simulink model "Copy_of_provaHITL_12_10_completosensori_BUONO"  (R2020b)
settings: Solver=FixedStepDiscrete  StartTime=0.0  StopTime=Inf  FixedStep=0.02  RelTol=1e-3  EnableMultiTasking=on
PostLoadFcn:
  | , if any(exist('dsrtsu_mdlpostloadfcn', 'file') == [2, 3, 6]), try dsrtsu_mdlpostloadfcn('Execute', bdroot); catch fprintf('Error in PostLoadFcn (dsrtsu_mdlpostloadfcn) for model "%s":\n %s\n', bdroot, lasterr); end, end,
InitFcn:
  | , if any(exist('rtifpga_mdlclblib', 'file') ~= 0), rtifpga_mdlclblib('Init', bdroot); end,
values from neighbouring files (symbols this model uses):
  attuatore_Amax = deg2rad(27)    [AVVIO_AENEA_DATA.m]    (also in workspace_SFT.mat = 0.349065850399)
  attuatore_Amin = deg2rad(-23)    [AVVIO_AENEA_DATA.m]
  attuatore_Emax = deg2rad(18)    [AVVIO_AENEA_DATA.m]    (also in workspace_SFT.mat = 0.436332312999)
  attuatore_Emin = deg2rad(-32)    [AVVIO_AENEA_DATA.m]
  attuatore_Rmax = deg2rad(30)    [AVVIO_AENEA_DATA.m]    (also in workspace_SFT.mat = 0.436332312999)
  attuatore_Rmin = deg2rad(-30)    [AVVIO_AENEA_DATA.m]
  attuatore_Tmax = 1    [AVVIO_AENEA_DATA.m]    (also in workspace_SFT.mat = 0.6)
  attuatore_Tmin = 0    [AVVIO_AENEA_DATA.m]    (also in workspace_SFT.mat)
  interventoA_05 = 6    [AVVIO_AENEA_DATA.m]    (also in workspace_SFT.mat)
  interventoA_1 = 2    [AVVIO_AENEA_DATA.m]    (also in workspace_SFT.mat)
  interventoE_05 = 7.5    [AVVIO_AENEA_DATA.m]    (also in workspace_SFT.mat)
  interventoE_1 = 3.2    [AVVIO_AENEA_DATA.m]    (also in workspace_SFT.mat)
  interventoT = 0.1    [AVVIO_AENEA_DATA.m]    (also in workspace_SFT.mat)
  inv_A = -1    [AVVIO_AENEA_DATA.m]
  inv_comp_h = -1    [AVVIO_AENEA_DATA.m]
  inv_E = 1    [AVVIO_AENEA_DATA.m]
  inv_R = 1    [AVVIO_AENEA_DATA.m]
  inv_T = 1    [AVVIO_AENEA_DATA.m]
  K_AW_B_AP_quota = 1000    [AVVIO_AENEA_DATA.m]
  K_AW_B_becc = -250    [AVVIO_AENEA_DATA.m]
  K_AW_B_imb = 0    [AVVIO_AENEA_DATA.m]
  K_AW_B_roll = 500    [AVVIO_AENEA_DATA.m]
  K_imb_inv = -0.001306    [AVVIO_AENEA_DATA.m]
  Kd_h_app = 0.085    [AVVIO_AENEA_DATA.m]
  Kd_h_flare = 0.01    [AVVIO_AENEA_DATA.m]
  Ki_AP_quota_select = 0.01936    [AVVIO_AENEA_DATA.m]
  Ki_AP_rotta = 0.002    [AVVIO_AENEA_DATA.m]
  Ki_AP_vel = 0.025175    [AVVIO_AENEA_DATA.m]
  Ki_becch = -0.1963    [AVVIO_AENEA_DATA.m]
  Ki_h_app = 0.055    [AVVIO_AENEA_DATA.m]
  Ki_h_cruise = 0.008    [AVVIO_AENEA_DATA.m]
  Ki_h_flare = 0.07    [AVVIO_AENEA_DATA.m]
  Ki_roll = 0.004528    [AVVIO_AENEA_DATA.m]
  Kp_AP_quota_hold_h = 0.5503    [AVVIO_AENEA_DATA.m]
  Kp_AP_quota_hold_l = 0.5503    [AVVIO_AENEA_DATA.m]
  Kp_AP_quota_select = 0.02647    [AVVIO_AENEA_DATA.m]
  Kp_AP_rotta = 0.520    (= 0.52)    [AVVIO_AENEA_DATA.m]
  Kp_AP_vel = 0.132175    [AVVIO_AENEA_DATA.m]
  Kp_becch = -0.30    (= -0.3)    [AVVIO_AENEA_DATA.m]
  Kp_comp_h = 0.035    [AVVIO_AENEA_DATA.m]
  Kp_h_app_max = 0.086    [AVVIO_AENEA_DATA.m]
  Kp_h_app_min = 0.01    [AVVIO_AENEA_DATA.m]
  Kp_h_cruise = 0.04    [AVVIO_AENEA_DATA.m]
  Kp_h_flare = 0.1    [AVVIO_AENEA_DATA.m]
  Kp_imb = 0.0019415    [AVVIO_AENEA_DATA.m]
  Kp_p = 0.006913    [AVVIO_AENEA_DATA.m]
  Kp_q = -0.025    [AVVIO_AENEA_DATA.m]
  Kp_roll = 0.0718    [AVVIO_AENEA_DATA.m]
  Kp_Rotta_ATO = 4    [AVVIO_AENEA_DATA.m]    (also in workspace_SFT.mat)
  phi_max = deg2rad(30)    [AVVIO_AENEA_DATA.m]
  phi_min = deg2rad(-30)    [AVVIO_AENEA_DATA.m]
  safe_phi = 55    [AVVIO_AENEA_DATA.m]    (also in workspace_SFT.mat)
  safe_V = 40    [AVVIO_AENEA_DATA.m]    (also in workspace_SFT.mat)
  t_AP = 0.02    [AVVIO_AENEA_DATA.m]    (also in workspace_SFT.mat)
  theta_max = deg2rad(15)    [AVVIO_AENEA_DATA.m]
  theta_min = deg2rad(-15)    [AVVIO_AENEA_DATA.m]
  time_alarm_SAFE = 1    [AVVIO_AENEA_DATA.m]    (also in workspace_SFT.mat)
  tsamp = 0.02    [workspace_SFT.mat]
  V_max = 30    [AVVIO_AENEA_DATA.m]
  V_stall = 11    [AVVIO_AENEA_DATA.m]
  vel_wp1_al = 25    [AVVIO_AENEA_DATA.m]    (also in workspace_SFT.mat)
  vel_wp2_al = 20    [AVVIO_AENEA_DATA.m]    (also in workspace_SFT.mat)
undefined symbols (not defined in the file or in its folder): DiscIntNeverNeededParam, Newton, Raphson
libraries: simulink_extras x33, arduinolib x20, pid_lib x8, svdutilitieslib x3, simulink x3, dspsigops x3, aerolibtransform2sys x2, aerolibtransform2 x2
(part 5 of 8)

== system Copy_of_provaHITL_12_10_completosensori_BUONO/AUTOPILOTA/CONTROLLI INTERNI E SWITCH1/Controllore PID/elevator - landing ==
  In1 : Inport
  Tas : Inport  Port=2
  AL : Inport  Port=3
  Constant5 : Constant  Value=0
  Multiport Switch2 : MultiPortSwitch  DataPortOrder=Zero-based contiguous  Inputs=2  zeroidx=on
  Switch1 : Switch  Threshold=16
  Out1 : Outport  VectorParamsAs1DForOutWhenUnconnected=off
  wires:
  Multiport Switch2/1 -> Out1/1
  Tas/1 -> Switch1/2
  In1/1 -> Multiport Switch2/2, Switch1/1
  AL/1 -> Multiport Switch2/1
  Constant5/1 -> Switch1/3
  Switch1/1 -> Multiport Switch2/3

== system Copy_of_provaHITL_12_10_completosensori_BUONO/AUTOPILOTA/CONTROLLI INTERNI E SWITCH1/Controllore PID/elevator - takeoff ==
  In1 : Inport
  Fase_ATO : Inport  Port=2
  ATO : Inport  Port=3
  eq_rot : Inport  Port=4
  Degrees to Radians : simulink_extras/Transformations/Degrees to Radians
  Multiport Switch1 : MultiPortSwitch  DataPortOrder=Zero-based contiguous  Inputs=5  zeroidx=on
  Multiport Switch2 : MultiPortSwitch  DataPortOrder=Zero-based contiguous  Inputs=2  zeroidx=on
  Out1 : Outport  VectorParamsAs1DForOutWhenUnconnected=off
  wires:
  ATO/1 -> Multiport Switch2/1
  In1/1 -> Multiport Switch1/6, Multiport Switch1/5, Multiport Switch2/2
  Multiport Switch2/1 -> Out1/1
  Multiport Switch1/1 -> Multiport Switch2/3
  Fase_ATO/1 -> Multiport Switch1/1
  eq_rot/1 -> Degrees to Radians/1
  Degrees to Radians/1 -> Multiport Switch1/4, Multiport Switch1/3, Multiport Switch1/2

== system Copy_of_provaHITL_12_10_completosensori_BUONO/AUTOPILOTA/GESTIONE AUTOPILOTI1/Interruttore_Intervento/Enabled Subsystem ==
  Time : Inport
  Enable : EnablePort
  Constant1 : Constant  Value=0
  Constant2 : Constant
  Switch : Switch  Criteria=u2 > Threshold  Threshold=2
  1/0 : Outport  VectorParamsAs1DForOutWhenUnconnected=off
  wires:
  Time/1 -> Switch/2
  Constant1/1 -> Switch/1
  Constant2/1 -> Switch/3
  Switch/1 -> 1/0/1

== system Copy_of_provaHITL_12_10_completosensori_BUONO/AUTOPILOTA/GESTIONE AUTOPILOTI1/Interruttore_Intervento/Resettable Subsystem ==
  Reset : ResetPort  DisableCoverage=on
  CLOCK : Subsystem
  Time : Outport  VectorParamsAs1DForOutWhenUnconnected=off
  wires:
  CLOCK/1(Time) -> Time/1

== system Copy_of_provaHITL_12_10_completosensori_BUONO/AUTOPILOTA/GESTIONE AUTOPILOTI1/Interruttore_Safe/Enabled Subsystem ==
  Time : Inport
  Enable : EnablePort
  Constant1 : Constant  Value=0
  Constant2 : Constant
  Switch : Switch  Criteria=u2 > Threshold  Threshold=2
  1/0 : Outport  VectorParamsAs1DForOutWhenUnconnected=off
  wires:
  Time/1 -> Switch/2
  Constant1/1 -> Switch/1
  Constant2/1 -> Switch/3
  Switch/1 -> 1/0/1

== system Copy_of_provaHITL_12_10_completosensori_BUONO/AUTOPILOTA/GESTIONE AUTOPILOTI1/Interruttore_Safe/Resettable Subsystem ==
  Reset : ResetPort  DisableCoverage=on
  CLOCK : Subsystem
  Time : Outport  VectorParamsAs1DForOutWhenUnconnected=off
  wires:
  CLOCK/1(Time) -> Time/1

== system Copy_of_provaHITL_12_10_completosensori_BUONO/AUTOPILOTA/GESTIONE AUTOPILOTI1/Intervento Manager/Alarm_Timing_0.5sec ==
  Intervento_IN : Inport
  "Enabled " : Subsystem  TreatAsAtomicUnit=on
  Resettable Subsystem : Subsystem  TreatAsAtomicUnit=on
  Alarm : Outport  VectorParamsAs1DForOutWhenUnconnected=off
  wires:
  Intervento_IN/1 -> Resettable Subsystem/Reset, "Enabled "/Enable
  Resettable Subsystem/1(Time) -> "Enabled "/1("Time ")
  "Enabled "/1(Alarm_Int) -> Alarm/1

== system Copy_of_provaHITL_12_10_completosensori_BUONO/AUTOPILOTA/GESTIONE AUTOPILOTI1/Intervento Manager/Alarm_Timing_1sec ==
  Intervento_IN : Inport
  "Enabled " : Subsystem  TreatAsAtomicUnit=on
  Resettable Subsystem : Subsystem  TreatAsAtomicUnit=on
  Alarm : Outport  VectorParamsAs1DForOutWhenUnconnected=off
  wires:
  Intervento_IN/1 -> Resettable Subsystem/Reset, "Enabled "/Enable
  Resettable Subsystem/1(Time) -> "Enabled "/1("Time ")
  "Enabled "/1(Alarm_Int) -> Alarm/1

== system Copy_of_provaHITL_12_10_completosensori_BUONO/AUTOPILOTA/GESTIONE AUTOPILOTI1/Safe Manager/Alarm_Timing ==
  Alarm_IN : Inport
  "Enabled " : Subsystem  TreatAsAtomicUnit=on
  Resettable Subsystem : Subsystem  TreatAsAtomicUnit=on
  Alarm : Outport  VectorParamsAs1DForOutWhenUnconnected=off
  wires:
  Alarm_IN/1 -> Resettable Subsystem/Reset, "Enabled "/Enable
  Resettable Subsystem/1(Time) -> "Enabled "/1("Time ")
  "Enabled "/1(Alarm Safe) -> Alarm/1

== system Copy_of_provaHITL_12_10_completosensori_BUONO/AUTOPILOTA/Subsystem1/Subsystem1/APPROACH ==
  dist : Inport
  h_g : Inport  Port=2
  x_g : Inport  Port=3
  V_ : Inport  Port=4
  Enable : EnablePort  ShowOutputPort=on
  Abs : Abs
  Atan : Trigonometry  Operator=atan
  Constant1 : Constant  Value=20  SampleTime=0.02
  Constant2 : Constant  SampleTime=0.02
  Constant3 : Constant  SampleTime=0.02
  Constant4 : Constant  Value=0  SampleTime=0.02
  Discrete-Time Integrator : DiscreteIntegrator  gainval=1  ExternalReset=rising  SampleTime=0.02  LimitOutput=on  UpperSaturationLimit=1  LowerSaturationLimit=0  ICPrevOutput=DiscIntNeverNeededParam  ICPrevScaledInput=DiscIntNeverNeededParam
  Divide : Product  Inputs=*/
  Gain : Gain  Gain=-1
  MATLAB Function : MATLAB Function  TreatAsAtomicUnit=on
  Multiply : Product
  Multiply1 : Product
  Mux : Mux
  Sum : Sum  Inputs=|+-
  Sum1 : Sum  Inputs=|+-
  Switch : Switch  Criteria=u2 > Threshold
  x_g0 : Constant  Value=-100  SampleTime=0.02
  h_ref : Outport  VectorParamsAs1DForOutWhenUnconnected=off
  V1 : Outport  Port=2  VectorParamsAs1DForOutWhenUnconnected=off
  flare_data : Outport  Port=3  VectorParamsAs1DForOutWhenUnconnected=off
  landing_abort : Outport  Port=4  VectorParamsAs1DForOutWhenUnconnected=off
  rc_ref_app : Outport  Port=5  VectorParamsAs1DForOutWhenUnconnected=off
  wires:
  Constant1/1 -> V1/1
  h_g/1 -> Divide/1
  Sum/1 -> Divide/2
  x_g/1 -> Sum/1
  Sum1/1 -> Gain/1
  Gain/1 -> Multiply/2
  dist/1 -> Sum1/1
  x_g0/1 -> Sum/2, MATLAB Function/3(xg0), Sum1/2
  Multiply/1 -> h_ref/1
  Mux/1 -> flare_data/1
  MATLAB Function/2(h_f_out) -> Mux/2
  MATLAB Function/1(x_f_out) -> Mux/1
  Abs/1 -> MATLAB Function/2(gamma)
  MATLAB Function/3(k_x_out) -> Mux/3
  MATLAB Function/4(h_c_out) -> Mux/4
  MATLAB Function/5(no_solution) -> landing_abort/1
  Constant2/1 -> Discrete-Time Integrator/1
  Constant3/1 -> Switch/1
  Enable/1 -> Discrete-Time Integrator/2
  Constant4/1 -> Switch/3
  Discrete-Time Integrator/1 -> Switch/2
  Switch/1 -> MATLAB Function/1(reset)
  V_/1 -> Multiply1/1
  Multiply1/1 -> rc_ref_app/1
  Divide/1 -> Multiply1/2, Multiply/1, Atan/1
  Atan/1 -> Abs/1

== system Copy_of_provaHITL_12_10_completosensori_BUONO/AUTOPILOTA/Subsystem1/Subsystem1/CREAZIONE_WAYPOINT  ==
  Lat_Home : Inport
  Long_Home : Inport  Port=2
  h_Home : Inport  Port=3
  psi_Home : Inport  Port=4
  AUTOLANDING_WAYPOINTS : MATLAB Function  TreatAsAtomicUnit=on
  Constant : Constant  Value=vel_wp1_al
  Constant1 : Constant  Value=vel_wp2_al
  MATLAB Function : MATLAB Function  TreatAsAtomicUnit=on
  Radians to Degrees : simulink_extras/Transformations/Radians to Degrees
  Radians to Degrees1 : simulink_extras/Transformations/Radians to Degrees
  alt waypoint virtuale : Constant  Value=[45 45 45]
  distance waypoints virtuale : Constant  Value=[-1000 -800 2000]
  WP_info : Outport  VectorParamsAs1DForOutWhenUnconnected=off
  WP_param : Outport  Port=2  VectorParamsAs1DForOutWhenUnconnected=off
  wires:
  alt waypoint virtuale/1 -> AUTOLANDING_WAYPOINTS/4(alt)
  distance waypoints virtuale/1 -> MATLAB Function/4(distance)
  Lat_Home/1 -> MATLAB Function/1(lat_ini)
  Long_Home/1 -> MATLAB Function/2(long_ini)
  psi_Home/1 -> MATLAB Function/3(heading)
  h_Home/1 -> AUTOLANDING_WAYPOINTS/3(h_Home)
  MATLAB Function/1(lat_end) -> Radians to Degrees/1
  MATLAB Function/2(long_end) -> Radians to Degrees1/1
  Radians to Degrees/1 -> AUTOLANDING_WAYPOINTS/1(Lat_Home)
  Radians to Degrees1/1 -> AUTOLANDING_WAYPOINTS/2(Long_Home)
  AUTOLANDING_WAYPOINTS/1(WP_info) -> WP_info/1
  AUTOLANDING_WAYPOINTS/2(WP_param) -> WP_param/1
  Constant/1 -> AUTOLANDING_WAYPOINTS/5(vel_wp1_al)
  Constant1/1 -> AUTOLANDING_WAYPOINTS/6(vel_wp2_al)

== system Copy_of_provaHITL_12_10_completosensori_BUONO/AUTOPILOTA/Subsystem1/Subsystem1/FLARE ==
  x_e : Inport
  flare_data : Inport  Port=2
  V_ : Inport  Port=3
  Enable : EnablePort
  Constant1 : Constant  Value=18  SampleTime=0.02
  Demux : Demux
  Exp : Math  SignedPower=on  SaturateOnIntegerOverflow=on
  Exp1 : Math  SignedPower=on  SaturateOnIntegerOverflow=on
  Gain : Gain  Gain=-1
  Gain1 : Gain  Gain=-1
  Gain2 : Gain  Gain=-1
  MATLAB Function : MATLAB Function  Commented=on  TreatAsAtomicUnit=on
  Multiply{,1..3} (4 alike) : Product
  Multiply4 : Product  Inputs=3
  Sum{,1,3..4} (4 alike) : Sum  Inputs=|+-
  Sum2 : Sum  Inputs=|++
  x_e1 : InportShadow
  Tas_ref1 : Outport  VectorParamsAs1DForOutWhenUnconnected=off
  h_ref : Outport  Port=2  VectorParamsAs1DForOutWhenUnconnected=off
  RC_ref : Outport  Port=3  VectorParamsAs1DForOutWhenUnconnected=off
  wires:
  MATLAB Function/1(rotta) -> ?
  Constant1/1 -> Tas_ref1/1
  x_e/1 -> Sum/1
  Sum/1 -> Multiply/1
  Multiply/1 -> Gain/1
  Gain/1 -> Exp/1
  Exp/1 -> Multiply1/1
  Sum1/1 -> Multiply1/2
  Multiply1/1 -> Sum2/1
  flare_data/1 -> Demux/1
  Sum2/1 -> h_ref/1
  Gain1/1 -> Exp1/1
  Demux/1 -> Sum3/2, Sum/2  "x_f"
  Demux/2 -> Sum4/1, Sum1/1  "h_f"
  x_e1/1 -> Sum3/1
  Exp1/1 -> Multiply3/1
  Gain2/1 -> RC_ref/1
  Demux/4 -> Sum4/2, Sum1/2, Sum2/2  "h_c"
  Multiply2/1 -> Gain1/1
  Sum3/1 -> Multiply2/1
  Demux/3 -> Multiply2/2, Multiply4/3, Multiply/2  "k_x"
  Multiply3/1 -> Gain2/1
  Sum4/1 -> Multiply4/1
  V_/1 -> Multiply4/2
  Multiply4/1 -> Multiply3/2

== system Copy_of_provaHITL_12_10_completosensori_BUONO/AUTOPILOTA/Subsystem1/Subsystem1/INSEGUIMENTO CENTRO PISTA ==
  y_e : Inport
  psi_home : Inport  Port=2
  Enable : EnablePort
  Gain1 : Gain
  PID Controller : pid_lib/PID Controller  Controller=PI  Form=Parallel  TimeDomain=Discrete-time  UseExternalTs=off  SampleTime=-1  IntegratorMethod=Forward Euler  FilterMethod=Forward Euler  ControllerParametersSource=external  P=1  I=1  D=0  UseFilter=on  N=100  TunerSelectOption=Transfer Function Based (PID Tuner App)  InitialConditionSource=internal  InitialConditionForIntegrator=0  InitialConditionForFilter=0  DifferentiatorICPrevScaledInput=0  ExternalReset=none  TrackingMode=off  Kt=1  LimitOutput=off  SatLimitsSource=internal  UpperSaturationLimit=inf  LowerSaturationLimit=-inf  LinearizeAsGain=on  AntiWindupMode=none  Kb=1  POutMin=[]  POutMax=[]  IOutMin=[]  IOutMax=[]  DOutMin=[]  DOutMax=[]  NOutMin=[]  NOutMax=[]  SumOutMin=[]  SumOutMax=[]  SaturationOutMin=[]  SaturationOutMax=[]  PParamMin=[]  PParamMax=[]  IParamMin=[]  IParamMax=[]  DParamMin=[]  DParamMax=[]  NParamMin=[]  NParamMax=[]  KbParamMin=[]  KbParamMax=[]  KtParamMin=[]  KtParamMax=[]  KbOutMin=[]  KbOutMax=[]  KtOutMin=[]  KtOutMax=[]  IntegratorOutMin=[]  IntegratorOutMax=[]  FilterOutMin=[]  FilterOutMax=[]  SumI1OutMin=[]  SumI1OutMax=[]  SumI2OutMin=[]  SumI2OutMax=[]  SumI3OutMin=[]  SumI3OutMax=[]  SumI4OutMin=[]  SumI4OutMax=[]  SumDOutMin=[]  SumDOutMax=[]  DifferentiatorOutMin=[]  DifferentiatorOutMax=[]  FilterDiffOutCoefMin=[]  FilterDiffOutCoefMax=[]  ReciprocalOutMin=[]  ReciprocalOutMax=[]  SumDenOutMin=[]  SumDenOutMax=[]  SumNumOutMin=[]  SumNumOutMax=[]  DivideOutMin=[]  DivideOutMax=[]  UdiffTsProdOutMin=[]  UdiffTsProdOutMax=[]  NTsProdOutMin=[]  NTsProdOutMax=[]  UintegralTsProdOutMin=[]  UintegralTsProdOutMax=[]  UngainTsProdOutMin=[]  UngainTsProdOutMax=[]  IntegratorContinuousStateAttributes=''  IntegratorStateMustResolveToSignalObject=off  IntegratorRTWStateStorageClass=Auto  FilterContinuousStateAttributes=''  FilterStateMustResolveToSignalObject=off  FilterRTWStateStorageClass=Auto  ParallelPVariant=ExternalParameters  IdealPVariant=Disabled  IVariant=ExternalParameters  DVariant=Disabled  IntegratorVariant=Discrete  SatVariant=Disabled  AWVariant=Passthrough  PCopyVariant=Disabled  TRVariant=Disabled  FdbkBlocksVariant=Forward  IdealPFdbkVariant=Disabled  SatFdbkVariant=Disabled  DerivativeFilterVariant=Disabled  NVariant=Disabled  NCopyVariant=Disabled_SignalSpec  FilterICVariant=Disabled  IntegratorICVariant=InternalICs  ExternalResetVariant=Disabled  TRSumVariant=Passthrough  SumFdbkVariant=Disabled  SumVariant=Sum_PI  TsampFilterVariant=InternalTs  TsampNgainVariant=Passthrough  TsampIntegralVariant=Passthrough  ExternalSaturationOutDataTypeStr=Inherit: Same as second input
  Radians to Degrees2 : simulink_extras/Transformations/Radians to Degrees
  Sum3 : Sum  Inputs=|+-
  psi ref gain : Constant  Value=0.0052  SampleTime=t_AP
  psi ref gain1 : Constant  Value=0.00052  SampleTime=t_AP
  psi_ref_landing : Outport  VectorParamsAs1DForOutWhenUnconnected=off
  wires:
  psi_home/1 -> [psi_home]
  y_e/1 -> Gain1/1
  Gain1/1 -> PID Controller/1
  psi ref gain/1 -> PID Controller/2
  [psi_home] -> Sum3/1
  Sum3/1 -> Radians to Degrees2/1
  Radians to Degrees2/1 -> psi_ref_landing/1
  psi ref gain1/1 -> PID Controller/3
  PID Controller/1 -> Sum3/2

== system Copy_of_provaHITL_12_10_completosensori_BUONO/AUTOPILOTA/Subsystem1/Subsystem1/LLA to Flat Earth ==
  latlong : Inport
  h : Inport  Port=2
  ground height : Inport  Port=3
  latlong_ref : Inport  Port=4
  psi_ref : Inport  Port=5
  Degrees to Radians : simulink_extras/Transformations/Degrees to Radians
  LatLong wrap : aerolibtransform2sys/LatLong wrap  SystemSampleTime=-1  VariantActivationTime=update diagram  Latency=0  AutoFrameSizeCalculation=off
      settings: SourceProductBaseCode=AE
  LatLong wrap LL0 : aerolibtransform2sys/LatLong wrap  SystemSampleTime=-1  VariantActivationTime=update diagram  Latency=0  AutoFrameSizeCalculation=off
      settings: SourceProductBaseCode=AE
  Mux : Mux  Inputs=3
  Subsystem1 : Subsystem
  Sum : Sum  Inputs=++|
  Sum1 : Sum  Inputs=|+-
  Ze2height : UnaryMinus
  initial_latg : Selector  InputPortWidth=2  IndexOptions=Index vector (dialog)  Indices=[1]  OutputSizes=1
  Xe : Outport  VectorParamsAs1DForOutWhenUnconnected=off
  wires:
  Degrees to Radians/1 -> Subsystem1/1(pos_rad)
  initial_latg/1 -> Subsystem1/2(mu)
  ground height/1 -> Sum/2
  LatLong wrap/1 -> Degrees to Radians/1
  LatLong wrap LL0/1 -> Sum1/2, initial_latg/1
  Sum1/1 -> LatLong wrap/1
  Ze2height/1 -> Mux/3  "Pz"
  Subsystem1/1(Px) -> Mux/1
  Subsystem1/2(Py) -> Mux/2
  Mux/1 -> Xe/1
  latlong_ref/1 -> LatLong wrap LL0/1
  Sum/1 -> Ze2height/1  "alt"
  h/1 -> Sum/1
  psi_ref/1 -> Subsystem1/3(psi_ref)
  latlong/1 -> Sum1/1

== system Copy_of_provaHITL_12_10_completosensori_BUONO/AIR TX/GPS/GPS_Venus/Subsystem2/Subsystem ==
  In1 : Inport
  Enable : EnablePort
  Complex to Real-Imag : ComplexToRealImag  Output=Real
  MATLAB Function : MATLAB Function  TreatAsAtomicUnit=on
  Memory : Memory  InheritSampleTime=on
  Mux : Mux  Inputs=9
  Outport : Outport  VectorParamsAs1DForOutWhenUnconnected=off
  mario : Outport  Port=2  VectorParamsAs1DForOutWhenUnconnected=off
  wires:
  MATLAB Function/2(Long) -> Mux/2  "Long"
  Memory/1 -> MATLAB Function/2(out_prec)
  MATLAB Function/8(h_mean_sea) -> Mux/8  "h_mean_sea"
  MATLAB Function/3(V) -> Mux/3  "hor_speed"
  MATLAB Function/1(Lat) -> Mux/1  "Lat"
  Mux/1 -> Complex to Real-Imag/1
  MATLAB Function/9(h_WGS84) -> Mux/9  "h_WGS85"
  MATLAB Function/5(heading) -> Mux/5  "heading"
  MATLAB Function/6(fix_mode) -> Mux/6  "fix_GPS"
  MATLAB Function/4(Magnetic_declination) -> Mux/4
  MATLAB Function/7(n_sat) -> Mux/7
  Complex to Real-Imag/1 -> Memory/1, Outport/1
  In1/1 -> MATLAB Function/1(messaggio)
  MATLAB Function/10(indice_dimario) -> mario/1

== system Copy_of_provaHITL_12_10_completosensori_BUONO/AUTOPILOTA/AUTOPILOTI1/CONTROLLORE DI VELOCITA'/throttle - landing/Enabled Subsystem ==
  Trigger : TriggerPort  VariantControl=Variant  PortDimensions=1
  Constant : Constant  Value=0
  Out1 : Outport  InitialOutput=[1]  VectorParamsAs1DForOutWhenUnconnected=off
  wires:
  Constant/1 -> Out1/1

== system Copy_of_provaHITL_12_10_completosensori_BUONO/AUTOPILOTA/GESTIONE AUTOPILOTI1/Interruttore_Intervento/Resettable Subsystem/CLOCK ==
  Constant4 : Constant  Value=t_AP  SampleTime=t_AP
  Memory : Memory  InheritSampleTime=on
  Sum : Sum  Inputs=|++
  Time : Outport  VectorParamsAs1DForOutWhenUnconnected=off
  wires:
  Memory/1 -> Sum/2
  Sum/1 -> Memory/1, Time/1
  Constant4/1 -> Sum/1

== system Copy_of_provaHITL_12_10_completosensori_BUONO/AUTOPILOTA/GESTIONE AUTOPILOTI1/Interruttore_Safe/Resettable Subsystem/CLOCK ==
  Constant4 : Constant  Value=t_AP  SampleTime=t_AP
  Memory : Memory  InheritSampleTime=on
  Sum : Sum  Inputs=|++
  Time : Outport  VectorParamsAs1DForOutWhenUnconnected=off
  wires:
  Memory/1 -> Sum/2
  Sum/1 -> Memory/1, Time/1
  Constant4/1 -> Sum/1

== system Copy_of_provaHITL_12_10_completosensori_BUONO/AUTOPILOTA/GESTIONE AUTOPILOTI1/Intervento Manager/Alarm_Timing_0.5sec/Enabled  ==
  "Time " : Inport
  Enable : EnablePort
  Constant : Constant
  Constant1 : Constant  Value=0
  Switch : Switch  Criteria=u2 > Threshold  Threshold=0.5
  Alarm_Int : Outport  OutputWhenDisabled=reset  InitialOutput=0  VectorParamsAs1DForOutWhenUnconnected=off
  wires:
  "Time "/1 -> Switch/2
  Constant/1 -> Switch/1
  Constant1/1 -> Switch/3
  Switch/1 -> Alarm_Int/1

== system Copy_of_provaHITL_12_10_completosensori_BUONO/AUTOPILOTA/GESTIONE AUTOPILOTI1/Intervento Manager/Alarm_Timing_0.5sec/Resettable Subsystem ==
  Reset : ResetPort  DisableCoverage=on
  CLOCK : Subsystem
  Time : Outport  VectorParamsAs1DForOutWhenUnconnected=off
  wires:
  CLOCK/1(Time) -> Time/1

== system Copy_of_provaHITL_12_10_completosensori_BUONO/AUTOPILOTA/GESTIONE AUTOPILOTI1/Intervento Manager/Alarm_Timing_1sec/Enabled  ==
  "Time " : Inport
  Enable : EnablePort
  Constant : Constant
  Constant1 : Constant  Value=0
  Switch : Switch  Criteria=u2 > Threshold  Threshold=1
  Alarm_Int : Outport  OutputWhenDisabled=reset  InitialOutput=0  VectorParamsAs1DForOutWhenUnconnected=off
  wires:
  "Time "/1 -> Switch/2
  Constant/1 -> Switch/1
  Constant1/1 -> Switch/3
  Switch/1 -> Alarm_Int/1

== system Copy_of_provaHITL_12_10_completosensori_BUONO/AUTOPILOTA/GESTIONE AUTOPILOTI1/Intervento Manager/Alarm_Timing_1sec/Resettable Subsystem ==
  Reset : ResetPort  DisableCoverage=on
  CLOCK : Subsystem
  Time : Outport  VectorParamsAs1DForOutWhenUnconnected=off
  wires:
  CLOCK/1(Time) -> Time/1

== system Copy_of_provaHITL_12_10_completosensori_BUONO/AUTOPILOTA/GESTIONE AUTOPILOTI1/Safe Manager/Alarm_Timing/Enabled  ==
  "Time " : Inport
  Enable : EnablePort
  Constant : Constant
  Constant1 : Constant  Value=0
  Switch : Switch  Criteria=u2 > Threshold  Threshold=time_alarm_SAFE
  Alarm Safe : Outport  OutputWhenDisabled=reset  InitialOutput=0  VectorParamsAs1DForOutWhenUnconnected=off
  wires:
  "Time "/1 -> Switch/2
  Constant/1 -> Switch/1
  Constant1/1 -> Switch/3
  Switch/1 -> Alarm Safe/1

== system Copy_of_provaHITL_12_10_completosensori_BUONO/AUTOPILOTA/GESTIONE AUTOPILOTI1/Safe Manager/Alarm_Timing/Resettable Subsystem ==
  Reset : ResetPort  DisableCoverage=on
  CLOCK : Subsystem
  Time : Outport  VectorParamsAs1DForOutWhenUnconnected=off
  wires:
  CLOCK/1(Time) -> Time/1

== system Copy_of_provaHITL_12_10_completosensori_BUONO/AUTOPILOTA/Subsystem1/Subsystem1/LLA to Flat Earth/Subsystem1 ==
  pos_rad : Inport
  mu : Inport  Port=2
  psi_ref : Inport  Port=3
  Demux : Demux  Outputs=2
  SinCos : Trigonometry  Operator=sincos
  Subsystem : Subsystem
  Sum2 : Sum  Inputs=|++
  Sum3 : Sum  Inputs=|-+
  dEast : Product  Inputs=/*  RndMeth=Zero
  dNorth : Product  Inputs=*/  RndMeth=Zero
  x*cos : Product  RndMeth=Zero
  x*sin : Product  RndMeth=Zero
  y*cos : Product  RndMeth=Zero
  y*sin : Product  RndMeth=Zero
  Px : Outport  VectorParamsAs1DForOutWhenUnconnected=off
  Py : Outport  Port=2  VectorParamsAs1DForOutWhenUnconnected=off
  wires:
  SinCos/1 -> y*sin/2, x*sin/2
  dNorth/1 -> x*cos/1, x*sin/1
  Sum2/1 -> Px/1  "Px"
  Demux/2 -> dEast/2
  x*cos/1 -> Sum2/1
  Subsystem/2(dEast) -> dEast/1
  psi_ref/1 -> SinCos/1
  Demux/1 -> dNorth/1
  dEast/1 -> y*sin/1, y*cos/1
  Sum3/1 -> Py/1  "Py"
  y*cos/1 -> Sum3/2
  y*sin/1 -> Sum2/2
  Subsystem/1(dNorth) -> dNorth/2
  SinCos/2 -> x*cos/2, y*cos/2
  pos_rad/1 -> Demux/1
  x*sin/1 -> Sum3/1
  mu/1 -> Subsystem/1(mu)

== system Copy_of_provaHITL_12_10_completosensori_BUONO/AUTOPILOTA/GESTIONE AUTOPILOTI1/Intervento Manager/Alarm_Timing_0.5sec/Resettable Subsystem/CLOCK ==
  Constant4 : Constant  Value=t_AP  SampleTime=t_AP
  Memory : Memory  InheritSampleTime=on
  Sum : Sum  Inputs=|++
  Time : Outport  VectorParamsAs1DForOutWhenUnconnected=off
  wires:
  Memory/1 -> Sum/2
  Sum/1 -> Memory/1, Time/1
  Constant4/1 -> Sum/1

== system Copy_of_provaHITL_12_10_completosensori_BUONO/AUTOPILOTA/GESTIONE AUTOPILOTI1/Intervento Manager/Alarm_Timing_1sec/Resettable Subsystem/CLOCK ==
  Constant4 : Constant  Value=t_AP  SampleTime=t_AP
  Memory : Memory  InheritSampleTime=on
  Sum : Sum  Inputs=|++
  Time : Outport  VectorParamsAs1DForOutWhenUnconnected=off
  wires:
  Memory/1 -> Sum/2
  Sum/1 -> Memory/1, Time/1
  Constant4/1 -> Sum/1

== system Copy_of_provaHITL_12_10_completosensori_BUONO/AUTOPILOTA/GESTIONE AUTOPILOTI1/Safe Manager/Alarm_Timing/Resettable Subsystem/CLOCK ==
  Constant4 : Constant  Value=t_AP  SampleTime=t_AP
  Memory : Memory  InheritSampleTime=on
  Sum : Sum  Inputs=|++
  Time : Outport  VectorParamsAs1DForOutWhenUnconnected=off
  wires:
  Memory/1 -> Sum/2
  Sum/1 -> Memory/1, Time/1
  Constant4/1 -> Sum/1

== system Copy_of_provaHITL_12_10_completosensori_BUONO/AUTOPILOTA/Subsystem1/Subsystem1/LLA to Flat Earth/Subsystem1/Subsystem ==
  mu : Inport
  Constant : Constant  SampleTime=0.02
  Constant1 : Constant  Value=6378137  SampleTime=0.02
  Constant2 : Constant  SampleTime=0.02
  Constant3 : Constant
  Degrees to Radians : simulink_extras/Transformations/Degrees to Radians
  Product1 : Product  Inputs=*/  RndMeth=Zero
  Product2 : Product  RndMeth=Zero
  Product3 : Product  Inputs=**/  RndMeth=Zero
  Product4 : Product  RndMeth=Zero
  Subsystem : Subsystem
  Subsystem1 : Subsystem
  Sum1 : Sum  Inputs=|+-
  Trigonometric Function : Trigonometry  Operator=cos
  Trigonometric Function1 : Trigonometry  Operator=atan2
  Trigonometric Function2 : Trigonometry  Operator=atan2
  denom : aerolibtransform2/LLA to Flat Earth/Subsystem/Find Radian//Distance/denom  SystemSampleTime=-1  VariantActivationTime=update diagram  Latency=0  AutoFrameSizeCalculation=off
      settings: SourceProductBaseCode=AE
  e^1 : aerolibtransform2/Geocentric to  Geodetic Latitude/e^4  Commented=on  SystemSampleTime=-1
      settings: SourceProductBaseCode=AE
  sqrt : Sqrt  AlgorithmType=Newton-Raphson  SaturateOnIntegerOverflow=on
  dNorth : Outport  VectorParamsAs1DForOutWhenUnconnected=off
  dEast : Outport  Port=2  VectorParamsAs1DForOutWhenUnconnected=off
  wires:
  Constant2/1 -> Trigonometric Function1/1
  Constant1/1 -> Product1/1
  Product4/1 -> Trigonometric Function2/2
  Trigonometric Function/1 -> Product4/2
  Product3/1 -> Trigonometric Function1/2  "Rm"
  Subsystem/1(e) -> Subsystem1/1(e)
  Constant3/1 -> Trigonometric Function2/1
  Trigonometric Function1/1 -> dNorth/1
  Trigonometric Function2/1 -> dEast/1
  Product1/1 -> Product3/1, Product4/1  "Rn"
  denom/1 -> Product3/3, sqrt/1
  mu/1 -> Degrees to Radians/1
  Sum1/1 -> Product3/2
  Subsystem1/1(eps) -> denom/1, Product2/1, Product2/2
  Degrees to Radians/1 -> denom/2, Trigonometric Function/1
  Constant/1 -> Sum1/1
  sqrt/1 -> Product1/2
  Product2/1 -> Sum1/2

== system Copy_of_provaHITL_12_10_completosensori_BUONO/AUTOPILOTA/Subsystem1/Subsystem1/LLA to Flat Earth/Subsystem1/Subsystem/Subsystem ==
  Constant : Constant  Value=1/298.257223563  SampleTime=0.02
  Sum : Sum  Inputs=-+
  f : Constant  SampleTime=0.02
  e : Outport  VectorParamsAs1DForOutWhenUnconnected=off
  wires:
  Constant/1 -> Sum/1
  f/1 -> Sum/2
  Sum/1 -> e/1

== system Copy_of_provaHITL_12_10_completosensori_BUONO/AUTOPILOTA/Subsystem1/Subsystem1/LLA to Flat Earth/Subsystem1/Subsystem/Subsystem1 ==
  e : Inport
  Constant4 : Constant
  Product : Product
  Sqrt : Sqrt  SaturateOnIntegerOverflow=on
  Sum : Sum  Inputs=+-
  eps : Outport
  wires:
  Product/1 -> Sum/2
  Sqrt/1 -> eps/1
  e/1 -> Product/2, Product/1
  Constant4/1 -> Sum/1
  Sum/1 -> Sqrt/1

== matlab function Copy_of_provaHITL_12_10_completosensori_BUONO/BMP_280/MATLAB Function ==
  data: rate_l_up output; Cal_alt input; P input; P_int input; P_refer output double; P_cal input; rate_l_dw output
function [rate_l_up, P_refer, rate_l_dw]  = fcn( Cal_alt, P,P_int,P_cal)
%#codegen

persistent P_ref rl_up rl_dw

if isempty(P_ref)
    
    P_ref = 101325;
    
end

if isempty(rl_up)
    
    rl_up = 300;
    
end

if isempty(rl_dw)
    
    rl_dw = -300;
    
end

if Cal_alt == 1
    
    P_ref = P;
 
end

if P_int == 1
   
   P_ref = P_cal; 
   rl_up = 20;
   rl_dw = -20;
    
end
    


P_refer = P_ref;

rate_l_up = rl_up;
rate_l_dw = rl_dw;

== matlab function Copy_of_provaHITL_12_10_completosensori_BUONO/AIR TX/GPS/GPS_Venus/Subsystem2/Create_message ==
  data: status output; byte_pack input; messaggio output
function [status,messaggio]  = LETTURA_NMEA(byte_pack)

persistent message counter start_found end_found

status = false;       %ho aggiunto questo
messaggio = uint8(zeros(1,80)) ;
pos_end = uint8(0) ;
M = uint8(length(byte_pack)) ;


if isempty(end_found) 
    end_found = false ;
end 
if isempty(start_found) 
     start_found = false ;
end 
if isempty (counter) 
    counter = uint8(0) ;
end 
if isempty(message)
     message = uint8(zeros(1,80)) ;
end



if start_found == 0 
    for i = uint8(1) : M  
        if byte_pack(i) == '$' 
            message(1:M - (i-1)) = byte_pack(i:end) ;
            counter = M - (i-1) ; 
            start_found = true ;
            break
        end
    end
    
    
elseif start_found == 1
    for i = uint8(1) : M  
        if byte_pack(i) == 13 
            end_found = true ;
            pos_end = i ;
            break
        end
    end
    
    if end_found == 1
        message(counter + 1 : counter + pos_end) = byte_pack(1:pos_end) ;
        status = true;       %ho aggiunto questo
        messaggio = message ;
        end_found = false ;
        counter = M - pos_end ;
        if pos_end == M 
            start_found = false ; 
            message = uint8(zeros(1,80)) ;
        else  
            start_found = true ;
            message(1:(M - pos_end)) = byte_pack(pos_end + 1 : end) ;
            message(M - pos_end +1 : 80) = ...
                uint8(zeros(1,80 - (M - pos_end) )) ;
        end
         

    else 
    message(counter + 1 : M + counter ) = byte_pack ;
    counter = M + counter  ;
   
    end
    
    
 
        
    
    
end

== matlab function Copy_of_provaHITL_12_10_completosensori_BUONO/AIR TX/GPS/GPS_Venus/Subsystem2/Subsystem/MATLAB Function ==
  data: messaggio input; Lat output; Long output; V output; Magnetic_declination output; heading output; fix_mode output; n_sat output; h_mean_sea output; h_WGS84 output; out_prec input; indice_dimario output
function [Lat,Long,V,Magnetic_declination,heading,fix_mode,n_sat,h_mean_sea,h_WGS84,indice_dimario] = parser_NMEA(messaggio,out_prec)
    

messaggio = char(messaggio) ;

comma_gga = uint8(zeros(1,14));
comma_rmc = uint8(zeros(1,12));
star = uint8(0);
dollar = uint8(0);
find_dollar = uint8(0);
find_comma = uint8(0);
message_type = uint8(zeros(1,5));
indice_dimario = uint8(0);





for i=1:length(messaggio)
   if messaggio(i) == '$'
       find_dollar = find_dollar + uint8(1);
   end
   if messaggio(i) == ','
       find_comma = find_comma + uint8(1);
   end
end
    
if (find_dollar == 1 && (find_comma == 12 || find_comma == 14))               % controllo se il numero di $ e , sono corretti all'interno di messaggio
                                                                             % altrimenti il messaggio è corrotto ed in output mando i messaggi
                                                                             % precedenti
dollar= find(messaggio == '$',1);

mess_type = messaggio(dollar(1) + 1 : dollar(1) + 5);                              % è il nome del messaggio arrivato

% decodifica mesaggio RMC

if mess_type == 'GPRMC'
comma_rmc = find(messaggio == ',');                                              % restituisce le posizioni delle virgole all'interno del messaggio
star = find(messaggio == '*');                                               % restituisce la posizione dell'asterisco all'interno del messaggio
dollar = find(messaggio == '$');                                             % restituisce la posizione del dollaro all'interno del messaggio

Lat_1 = str2double(messaggio(comma_rmc(3) + 1 : comma_rmc(3) + 2));
Lat_2 = str2double(messaggio(comma_rmc(3) + 3 : comma_rmc(4) - 1))/60;
Lat = Lat_1 + Lat_2;
if messaggio(comma_rmc(4) + 1) == 'S'
Lat = -Lat; 
end

Long_1 = str2double(messaggio(comma_rmc(5) + 1 : comma_rmc(5) + 3));
Long_2 = str2double(messaggio(comma_rmc(5) + 4 : comma_rmc(6) - 1))/60;
Long = Long_1 + Long_2;
if messaggio(comma_rmc(6) + 1) == 'W'
Long = -Long; 
end

V = str2double(messaggio(comma_rmc(7) + 1 : comma_rmc(8) - 1)); 
    
heading = str2double(messaggio(comma_rmc(8) + 1 : comma_rmc(9) - 1));

Magnetic_declination = str2double(messaggio(comma_rmc(10) + 1 : comma_rmc(11) - 1));
if messaggio(comma_rmc(11) + 1) == 'W'
Magnetic_declination = -Magnetic_declination; 
end

% questi dati non sono presenti nel messaggio rmc, quindi prendo quelli
% precedenti

fix_mode = complex(out_prec(6),0);

n_sat = complex(out_prec(7),0) ;

h_mean_sea = complex(out_prec(8),0) ;

h_WGS84 = complex(out_prec(9),0) ;


%%%%%%%%%%%%%%%%%%%%%%%%%%%%%%%%%%%%%%%%%%%%%%%%%%%%%%%%%

% calcolo checksum

ck_ric = char(zeros(1,2)) ;
ck_ric(1) = messaggio(star(1) + uint8(1))  ;
ck_ric(2) = messaggio(star(1) + uint8(2)) ;

NMEA_rmc_string = uint8(messaggio(dollar(1)+1:star(1)-1)) ;

checksum = uint8(0) ;
for i = 1:length(NMEA_rmc_string) 
    checksum = bitxor(checksum,NMEA_rmc_string(i),'uint8') ;
end

if checksum ~= hex2dec(ck_ric) 
    Lat = out_prec(1) ;
    Long = out_prec(2) ;
    V = out_prec(3) ;
    Magnetic_declination = out_prec(4);
    heading = out_prec(5) ; 
    fix_mode = complex(out_prec(6),0);
    n_sat = complex(out_prec(7),0) ;
    h_mean_sea = complex(out_prec(8),0) ;
    h_WGS84 = complex(out_prec(9),0) ;
    indice_dimario = uint8(10);
end

%%%%%%%%%%%%%%%%%%%%%%%%%%%%%%%%%%%%%%%%%%%%%%%%%%%%%%%%%%%

% decodifica mesaggio GGA

elseif mess_type == 'GPGGA'
comma_gga = find(messaggio == ','); 
star = find(messaggio == '*');
dollar = find(messaggio == '$');


Lat_1 = str2double(messaggio(comma_gga(2) + 1 : comma_gga(2) + 2));
Lat_2 = str2double(messaggio(comma_gga(2) + 3 : comma_gga(3) - 1))/60;
Lat = Lat_1 + Lat_2;
if messaggio(comma_gga(3) + 1) == 'S'
Lat = -Lat; 
end


Long_1 = str2double(messaggio(comma_gga(4) + 1 : comma_gga(4) + 3));
Long_2 = str2double(messaggio(comma_gga(4) + 4 : comma_gga(5) - 1))/60;
Long = Long_1 + Long_2;
if messaggio(comma_gga(5) + 1) == 'W'
Long = -Long; 
end


fix_mode = str2double(messaggio(comma_gga(6) + 1)); 

n_sat = str2double(messaggio(comma_gga(7) + 1 : comma_gga(8) - 1));

h_mean_sea = str2double(messaggio(comma_gga(9) + 1 : comma_gga(10) - 1));

h_WGS84 = str2double(messaggio(comma_gga(11) + 1 : comma_gga(12) - 1));

% questi dati non sono presenti nel messaggio rmc, quindi prendo quelli
% precedenti

V = out_prec(3) ;

Magnetic_declination = out_prec(4);

heading = out_prec(5) ; 

%%%%%%%%%%%%%%%%%%%%%%%%%%%%%%%%%%%%%%%%%%%%%%%%%%%%%%%%%%%%%%%%%%%

% calcolo del checksum
ck_ric = char(zeros(1,2)) ;
ck_ric(1) = messaggio(star(1) + uint8(1))  ;
ck_ric(2) = messaggio(star(1) + uint8(2)) ;

NMEA_gga_string = uint8(messaggio(dollar(1)+1:star(1)-1)) ;

checksum = uint8(0) ;
for i = 1:length(NMEA_gga_string) 
    checksum = bitxor(checksum,NMEA_gga_string(i),'uint8') ;
end

if checksum ~= hex2dec(ck_ric) 
    Lat = out_prec(1) ;
    Long = out_prec(2) ;
    V = out_prec(3) ;
    Magnetic_declination = out_prec(4);
    heading = out_prec(5) ; 
fix_mode = complex(out_prec(6),0);

n_sat = complex(out_prec(7),0) ;

h_mean_sea = complex(out_prec(8),0) ;

h_WGS84 = complex(out_prec(9),0) ;
indice_dimario = uint8(20);
   
    
end

%%%%%%%%%%%%%%%%%%%%%%%%%%%%%%%%%%%%%%%%%%%%%%%%%%%%%%%%%%%%%%%%%%%%
        
else
    
    Lat = out_prec(1) ;
    Long = out_prec(2) ;
    V = out_prec(3) ;
    Magnetic_declination = out_prec(4);
    heading = out_prec(5) ; 
fix_mode = complex(out_prec(6),0);

n_sat = complex(out_prec(7),0) ;

h_mean_sea = complex(out_prec(8),0) ;

h_WGS84 = complex(out_prec(9),0) ; 
   
    
    
end


else
    
    Lat = out_prec(1) ;
    Long = out_prec(2) ;
    V = out_prec(3) ;
    Magnetic_declination = out_prec(4);
    heading = out_prec(5) ; 
    fix_mode = complex(out_prec(6),0);
    n_sat = complex(out_prec(7),0) ;
    h_mean_sea = complex(out_prec(8),0) ;
    h_WGS84 = complex(out_prec(9),0) ; 
end

end

== stateflow chart Copy_of_provaHITL_12_10_completosensori_BUONO/AUTOPILOTA/Subsystem1/DECOLLO AUTOMATICO/Chart1 ==
  state Fase_0_ATO
    du:
    Fase_ATO = 0;
    psi_ref_selector = 0;
    theta_ground_selector = 0;
    psi_ref = 0;
    phi_ref = 0;
    eq_rot = 0;
    Tas_ref = 0;
    pitch_ref = 0;
    h_ref = 0;
  state Fase_2_ATO %rullaggio
    du:
    Fase_ATO = 2;
    % devo mettere uno switch sulla manetta che tramite FASE_ATO la incrementa gradualmente fino al massimo e poi switcho sul controllore di velocita
    psi_ref_selector=0;
    psi_ref = psi_hold;
    phi_ref = 0;
    h_ref = 0;
    eq_rot = 2;
    Tas_ref = 25;
  note: la condizione V_>10 va messa soltanto in HIL, altrimenti in presenza di vento simulato l'aereo non parte
  state Fase_1_ATO
    du:
    Fase_ATO = 1;
    manetta_ref = 0.1;
    psi_ref_selector=0;
    h_ref = 0;
    psi_ref = psi_hold;
    phi_ref = 0;
    eq_rot = 2;
  state Fase_3_ATO  %rotazione
    du:
    Fase_ATO = 3;
    psi_ref_selector=0;
    theta_ground_selector = 0;
    psi_ref = psi_hold;
    phi_ref = 0;
    h_ref = 0;
    pitch_ref = 10 + theta_ground_hold;
    Tas_ref = 25;
    %devo passare al controllore di pitch, prima davo direttamente l'angolo dell'equilibratore a picchiare (ora devo fare la rotazione)
  note: quando si carica su arduino mettere manetta_ref = 0.05
      | o leggermente piu alto, in modo che l'elica giri ma non spinga
  state Fase_4_ATO  %salita
    du:
    Fase_ATO = 4;
    psi_ref_selector=0;
    psi_ref = psi_hold;
    h_ref = 35;
    RC_ref = 3;
    Tas_ref = 25;
    %devo passare al controllore di quota, prima controllavo il pitch
    %devo passare al controllore di roll canonico, prima fissavo il riferimento di roll = 0
  (default) -> Fase_0_ATO
  Fase_0_ATO -> Fase_1_ATO : [modo==3]{psi_ref_selector=1;}
  Fase_2_ATO %rullaggio -> Fase_3_ATO  %rotazione : [TAS >= 18 && V_ >= 10]{theta_ground_selector = 1;}
  Fase_1_ATO -> Fase_2_ATO %rullaggio : after(250,tick)
  Fase_3_ATO  %rotazione -> Fase_4_ATO  %salita : [h >= 2]
  Fase_4_ATO  %salita -> (junction 67)
  data: modo input; Fase_ATO output; manetta_ref output; psi_ref output; eq_rot output; phi_ref output; TAS input; pitch_ref output; h_ref output; Tas_ref output; h input; psi_hold input; RC_ref output; psi_ref_selector output; theta_ground_selector output; theta_ground_hold input; V_ input

== matlab function Copy_of_provaHITL_12_10_completosensori_BUONO/AUTOPILOTA/Subsystem1/Subsystem1/APPROACH/MATLAB Function ==
  data: reset input; gamma input; x_f_out output; h_f_out output; xg0 input; k_x_out output; h_c_out output; no_solution output
function [x_f_out,h_f_out,k_x_out,h_c_out,no_solution] = fcn(reset,gamma,xg0)

 

x_f=-200;
h_f=1.5;
%x_f=-300;
%h_f=10;
k_x=0.01;
h_c=-2;
x_td=5;
h_td_dot=-0.1;
x_td_dot=18;
no_solution = 0;

% x_f=-200;
% h_f=5;
% %x_f=-300;
% %h_f=10;
% k_x=0.01;
% h_c=-1;
% x_td=50;
% h_td_dot=-0.15;
% x_td_dot=18;
% no_solution = 0;

% F = [f(x_f,h_f,gamma,xg0); g(h_c,h_f,k_x,gamma); r(h_c,h_f,k_x,x_f,x_td); s(h_c,h_f,k_x,x_f,x_td,h_td_dot,x_td_dot)];
% 
% J = [ df1() df2(gamma) df3() df4();
%       dg1(k_x) dg2() dg3(h_f,h_c) dg4(k_x);
%       dr1(k_x,x_td,x_f) dr2(k_x,x_td,x_f) dr3(k_x,x_td,x_f,h_f,h_c) dr4();
%       ds1(k_x,x_td,x_f,x_td_dot) ds2(k_x,x_td,x_f,x_td_dot,h_f,h_c) ds3(k_x,x_td,x_f,x_td_dot,h_f,h_c) ds4(k_x,x_td,x_f,x_td_dot)]

persistent x x_new cycle_count eps

if (isempty(x) ||  reset == 0)
x = [h_f; x_f; k_x; h_c];
end

if (isempty(x_new) || reset == 0)
x_new = zeros(4,1);
end

if (isempty(eps) || reset == 0)
eps = ones(1,4);
end
   
if (isempty(cycle_count) || reset == 0)
cycle_count = 0;
end




while ~ (eps(1) < 0.1 && eps(2) < 0.1 && eps(3) < 0.1 && eps(4) < 0.1 )

F = [f(x(2),x(1),gamma,xg0); g(x(4),x(1),x(3),gamma); r(x(4),x(1),x(3),x(2),x_td); s(x(4),x(1),x(3),x(2),x_td,h_td_dot,x_td_dot)];

J = [ df1() df2(gamma) df3() df4();
      dg1(x(3)) dg2() dg3(x(1),x(4)) dg4(x(3));
      dr1(x(3),x_td,x(2)) dr2(x(3),x_td,x(2),x(1),x(4)) dr3(x(3),x_td,x(2),x(1),x(4)) dr4();
      ds1(x(3),x_td,x(2),x_td_dot) ds2(x(3),x_td,x(2),x_td_dot,x(1),x(4)) ds3(x(3),x_td,x(2),x_td_dot,x(1),x(4)) ds4(x(3),x_td,x(2),x_td_dot)] ; 
  
  
x_new = x - J^(-1)*F;

eps(1) = abs(x_new(1)-x(1));
eps(2) = abs(x_new(2)-x(2));
eps(3) = abs(x_new(3)-x(3));
eps(4) = abs(x_new(4)-x(4));


x = x_new;

cycle_count = cycle_count + 1;

if cycle_count > 10
   no_solution = 1; 
   break; 
end

end

if (eps(1) < 0.1 && eps(2) < 0.1 && eps(3) < 0.1 && eps(4) < 0.1 )
   
h_f_out = x(1);
x_f_out = x(2);
k_x_out = x(3);
h_c_out = x(4);

else
    
h_f_out = 0;
x_f_out = 0;
k_x_out = 0;
h_c_out = 0;    
end

function y = f(x_f,h_f,gamma,xg0)                 %inizio equazioni sistema non lineare
y = h_f+(x_f-xg0)*tan(gamma);
end

function y = g(h_c,h_f,k_x,gamma)
y = (h_f-h_c)*k_x-tan(gamma);
end

function y = r(h_c,h_f,k_x,x_f,x_td)
y = h_c + (h_f-h_c)*exp(-k_x*(x_td-x_f));
end

function y = s(h_c,h_f,k_x,x_f,x_td,h_td_dot,x_td_dot)
y = h_td_dot + (h_f-h_c)*k_x*x_td_dot*exp(-k_x*(x_td-x_f));        
end                                                                   % fine equazioni sistema non lineare

function y = df1()                                                    %inizio derivate
y = 1;
end

function y = df2(gamma)
y = tan(gamma);
end

function y = df3()
y = 0;
end

function y = df4()
y = 0;
end

function y = dg1(k_x)
y = k_x;
end

function y = dg2()
y = 0;
end

function y = dg3(h_f,h_c)
y = h_f-h_c;
end

function y = dg4(k_x)
y = -k_x;
end

function y = dr1(k_x,x_td,x_f)
y = exp(-k_x*(x_td-x_f));
end

function y = dr2(k_x,x_td,x_f,h_f,h_c)
y = (h_f-h_c)*k_x*exp(-k_x*(x_td-x_f));
end

function y = dr3(k_x,x_td,x_f,h_f,h_c)
y = (h_f-h_c)*(x_f-x_td)*exp(-k_x*(x_td-x_f));
end

function y = dr4()
y = 1;
end

function y = ds1(k_x,x_td,x_f,x_td_dot)
y = k_x*x_td_dot*exp(-k_x*(x_td-x_f));
end

function y = ds2(k_x,x_td,x_f,x_td_dot,h_f,h_c)
y = (h_f-h_c)*k_x^2*x_td_dot*exp(-k_x*(x_td-x_f));
end

function y = ds3(k_x,x_td,x_f,x_td_dot,h_f,h_c)
y = (h_f-h_c)*x_td_dot*exp(-k_x*(x_td-x_f))+(h_f-h_c)*k_x*x_td_dot*(x_f-x_td)*exp(-k_x*(x_td-x_f));
end

function y = ds4(k_x,x_td,x_f,x_td_dot)
y = -k_x*x_td_dot*exp(-k_x*(x_td-x_f));
end



end

== matlab function Copy_of_provaHITL_12_10_completosensori_BUONO/AUTOPILOTA/Subsystem1/Subsystem1/CALIBRATING_HOME_COORDINATES ==
  data: Cal_home input; Lat_Home output; Long_Home output; Lat input; Long input; h input; psi input; h_Home output; psi_Home output; GC_info input; WP_AL input; WP_db_info input
function [Lat_Home,Long_Home,h_Home,psi_Home] = fcn(Cal_home,Lat,Long,h,psi,GC_info,WP_AL,WP_db_info)
%#codegen

persistent Lat_H;
persistent Long_H;
persistent h_H;
persistent psi_H;
persistent counter;

if isempty( Lat_H)
    Lat_H = 0;
end

if isempty(Long_H)
   Long_H = 0;
end

if isempty(h_H)
    h_H = 0;
end

if isempty(psi_H)
    psi_H = 2.8274;        %162deg      (%2.79-160deg)
end

if isempty(counter)
    counter = 1;
end




% if Cal_home(1)==1
%     
%     Lat_H = Lat;
%     Long_H = Long;
%     h_H = h;
%     psi_H = psi;
%     
% end
% 
% if GC_info == 3
%     counter = 1;
%     for indice=1:size(WP_AL,1)
%         if WP_db_info(indice,5)==1
%             counter=indice;
%         end
%     end
% end
% 
% AL = WP_AL(counter,2);
% LatWP = WP_AL(counter,5);
% LongWP = WP_AL(counter,6);
% 
% LatWP2 = WP_AL(counter+1,5);
% LongWP2 = WP_AL(counter+1,6);    
% 
% dr=pi/180;
% 
% if AL == 1
%     Lat_Home = LatWP*dr;
%     Long_Home = LongWP*dr;
%     h_Home = WP_AL(counter,7);
%     psi_Home = atan2(sin(LongWP2*dr-LongWP*dr)*cos(LatWP2*dr),cos(LatWP*dr)*sin(LatWP2*dr)-sin(LatWP*dr)*cos(LatWP2*dr)*cos(LongWP2*dr-LongWP*dr));
% else
%     Lat_Home=Lat_H;
%     Long_Home=Long_H;
%     h_Home=h_H;
%     psi_Home=psi_H;
% end
dr=pi/180;

LatWP = WP_AL(1,5);
LongWP = WP_AL(1,6);

LatWP2 = WP_AL(2,5);
LongWP2 = WP_AL(2,6); 

Lat_Home = LatWP*dr;
Long_Home = LongWP*dr;
h_Home = WP_AL(1,7);
psi_Home = atan2(sin(LongWP2*dr-LongWP*dr)*cos(LatWP2*dr),cos(LatWP*dr)*sin(LatWP2*dr)-sin(LatWP*dr)*cos(LatWP2*dr)*cos(LongWP2*dr-LongWP*dr));

if psi_Home < 0
    psi_Home = 2*pi - abs(psi_Home);
end

== stateflow chart Copy_of_provaHITL_12_10_completosensori_BUONO/AIR TX/Enable /Chart ==
  state sendbyte(bt,n) [function]
  state Inputblock
    entry: i=1;
    Inputblock -> (junction 28)
    (junction 32) -> (junction 28) [order 1] : [ i<Len]
        | {i++;}
    (junction 28) -> (junction 32) : {sendbyte(datain,i);}
    (junction 32) -> (junction 48) [order 2] : {i=1;}
  (default) -> Inputblock
  data: bt function_input uint8; n function_input; datain input uint8; Len input uint16 size=1; i local uint8 =0

== matlab function Copy_of_provaHITL_12_10_completosensori_BUONO/AUTOPILOTA/Subsystem1/Subsystem1/CREAZIONE_WAYPOINT /MATLAB Function ==
  data: lat_end output; long_end output; lat_ini input; long_ini input; heading input; distance input


function [lat_end,long_end] = fcn2(lat_ini,long_ini,heading,distance)


lat_end=zeros(1,3);
long_end=zeros(1,3);

R=6378137 ; %Earth Radius  

for n=1:3
    
lat_end(n) = asin(sin(lat_ini)*cos(distance(n)/R) + cos(lat_ini)*sin(distance(n)/R)*cos(heading));
long_end(n) = long_ini + atan2(sin(heading)*sin(distance(n)/R)*cos(lat_ini), cos(distance(n)/R)-sin(lat_ini)*sin(lat_end(n))); 


end


end

== matlab function Copy_of_provaHITL_12_10_completosensori_BUONO/AIR TX/Heartbeat/Alarm set ==
  data: Alarm input; H_mav output; Rx_mode input

%%

function H_mav = Allarm_set(Alarm, Rx_mode)
%#cambia lo stato se c'è un allarme attivo
% Allarm: possibili allarmi proveniente dall'autopilota
% Rx_mode: richiesta da parte della stazione di terra
% H_mav: setto i parametri Base_mode e System_status del Heartbeat


H_mav = uint8(Rx_mode); % setta la modalità con quella ricevuta da terra

% se un allarme si attiva ha la precedenza sulla richiesta della QGC

if Alarm(1) == 1 % ovvero l'aereo è entrato in safe e si pone su traettoria circolare di sicurezza
    
    H_mav(1) = uint8(220); % MAV_MODE_AUTO_ARMED
    H_mav(2) = uint8(5);   % MAV_STATE_CRITICAL
%     H_mav(3) = uint8(128); % MAV_MODE_FLAG_SAFETY_ARMED

end

% se l'allareme di intervento pilota è attivo ha precedenza sull'allarm
% sefe per cui bisogna riscrivere lo stato del pilota

if Alarm(2) == 1 % si è attivato l'allarme dell'intervento pilota 
    
    H_mav(1) = uint8(216); % MAV_MODE_GUIDED_ARMED
    H_mav(2) = uint8(4);   % MAV_STATE_ACTIVE
%     H_mav(3) = uint8(8);   % MAV_MODE_FLAG_GUIDED_ENABLED

end

== matlab function Copy_of_provaHITL_12_10_completosensori_BUONO/AIR TX/If_subsystem/iflogic_function ==
  data: H50 input; iflogic output; H10 input
function iflogic = fcn(H50,H10)
%#codegen
% prende in ingeresso i counter che contano il tempo
% e dice quale messaggio bisogna inviare in base alle frequenze scelte in
% Heartbeat:            1Hz
% SCALED_IMU:           20Hz
%attitude:              20Hz
%GLOBAL_POSITION_INT:   1Hz
%SYS_STATUS:            3Hz
%VFR_HUD:               2Hz
%SERVO_OUTPUT_RAW       1Hz
%SCALED_PRESSURE        1Hz

if H50 == 1  || H50==3
    iflogic=uint8(26); % SCALED_IMU 20Hz
elseif H50==2 || H50==4
    iflogic=uint8(30); %attitude 20Hz
elseif  H50==0 && H10==2
    iflogic=uint8(33); %GLOBAL_POSITION_INT 1Hz
elseif  H50==0 && H10==6
    iflogic=uint8(34); %GLOBAL_POSITION_INT_RAW 1Hz
elseif  H50==0 && H10==0
    iflogic=uint8(0); %Heartbeat 1Hz
elseif H50==0 && (H10==1 || H10==5 || H10==9)
    iflogic=uint8(1); %SYS_STATUS 3Hz
elseif H50==0 && (H10==3 || H10==8)
    iflogic=uint8(74); %VFR_HUD 2Hz
elseif H50==0 && (H10==7)
    iflogic=uint8(36); %SERVO_OUTPUT_RAW 1Hz
elseif H50==0 && (H10==4)
    iflogic=uint8(29); %SCALED_PRESSURE 1Hz
else
    iflogic=uint8(255); %non esiste nessun messaggio con questo codice
    
end
